simulink model "raspberrypi_multicore_audio_tasks_mapped"  (R2021a)
settings: Solver=FixedStepAuto  StartTime=0.0  StopTime=10.0  RelTol=1e-3  EnableMultiTasking=on
undefined symbols (not defined in the file): plughw
libraries: audiofilters x3, raspberrypiAVlib x2, dspindex x1, audiodynamicrange x1
settings Model: ExplicitPartitioning=on  Creator=The MathWorks, Inc.  LastModifiedBy=The MathWorks, Inc.
settings SolverCC: ConcurrentTasks=on  AlgebraicLoopSolver=TrustRegion  PositivePriorityOrder=on  AutoInsertRateTranBlk=on  InsertRTBMode=Never (minimum delay)
settings OptimizationCC: EnhancedBackFolding=on  PassReuseOutputArgsAs=Individual arguments  ZeroExternalMemoryAtStartup=off  ZeroInternalMemoryAtStartup=off  MaxStackSize=64  OptimizeBlockOrder=speed  DifferentSizesBufferReuse=on  OptimizationCustomize=off  EfficientTunableParamExpr=on
settings DebuggingCC: ParameterTunabilityLossMsg=error  SFMachineParentedDataDiag=warning
settings HardwareCC: ProdBitPerPointer=32  ProdBitPerSizeT=32  ProdBitPerPtrDiffT=32  ProdLargestAtomicInteger=Long  ProdLargestAtomicFloat=Double  ProdWordSize=32  ProdLongLongMode=on  ProdHWDeviceType=ARM Compatible->ARM Cortex
settings RTWCC: SystemTargetFile=ert.tlc  HardwareBoard=Raspberry Pi  TLCOptions="-aInlineSetEventsForThisBaseRateFcn=TLC_FALSE -aSuppressMultiTaskScheduler=TLC_FALSE  -aRateBasedStepFcn=0"  TemplateMakefile=ert_default_tmf  Toolchain=GNU GCC Embedded Linux  BuildConfiguration=Faster Runs
settings CodeAppCC: ForceParamTrailComments=on  IgnoreCustomStorageClasses=off  OperatorAnnotations=on  SimulinkDataObjDesc=on  SFDataObjDesc=on  InsertBlockDesc=on
settings ERTTargetCC: SupportVariableSizeSignals=on

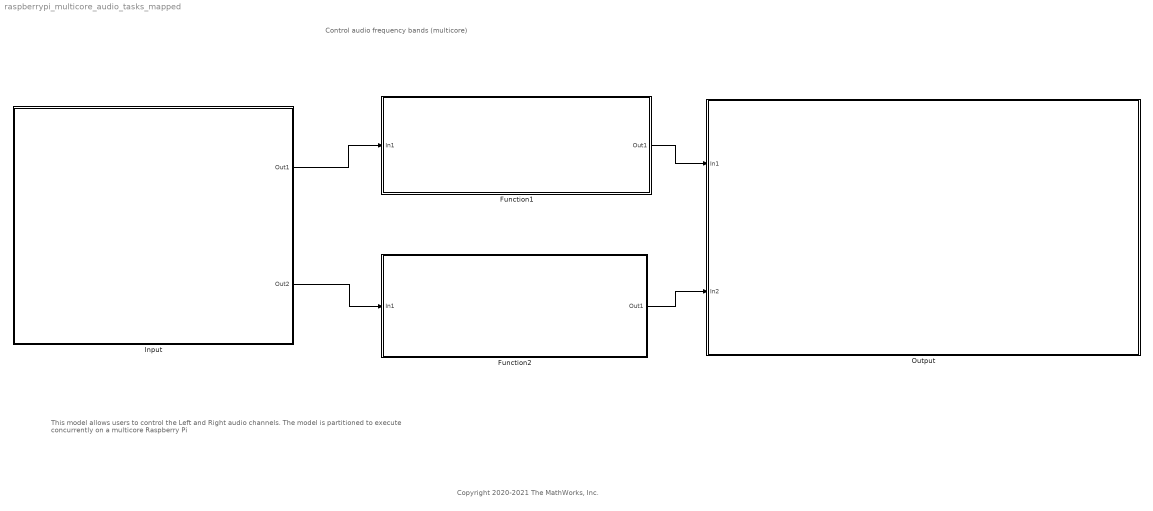
== system raspberrypi_multicore_audio_tasks_mapped ==
  note: This model allows users to control the Left and Right audio channels. The model is partitioned to execute concurrently on a multicore Raspberry Pi
  note: Copyright 2020-2021 The MathWorks, Inc.
  note: Control audio frequency bands (multicore)
  Function1 : Subsystem  TreatAsAtomicUnit=on
  Function2 : Subsystem  TreatAsAtomicUnit=on
  Input : Subsystem  TreatAsAtomicUnit=on
  Output : Subsystem  TreatAsAtomicUnit=on
  wires:
  Input/1(Out1) -> Function1/1(In1)
  Input/2(Out2) -> Function2/1(In1)
  Function1/1(Out1) -> Output/1(In1)
  Function2/1(Out1) -> Output/2(In2)

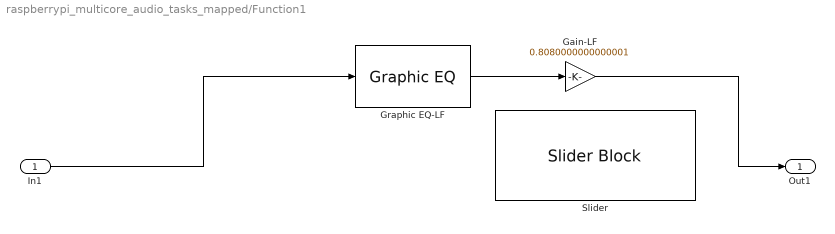
== system raspberrypi_multicore_audio_tasks_mapped/Function1 ==
  In1 : Inport
  Gain-LF : Gain  Gain=0.8080000000000001  OutDataTypeStr=single
  Graphic EQ-LF : audiofilters/Graphic EQ  EQOrder=2  Bandwidth=2/3 octave  Structure=Cascade  Gain_25=12  Gain_31_5=16  Gain_40=16  Gain_50=0  Gain_63=12  Gain_80=0  Gain_100=12  Gain_125=16  Gain_160=12  Gain_200=0  Gain_250=12  Gain_315=-1.200  Gain_400=10.800  Gain_500=6  Gain_630=6  Gain_800=0  Gain_1000=5  Gain_1250=0  Gain_1600=6  Gain_2000=6  Gain_2500=6  Gain_3150=0  Gain_4000=-20  Gain_5000=0  Gain_6300=-20  Gain_8000=-20  Gain_10000=-20  Gain_12500=0  Gain_16000=-20  Gain_20000=0  InheritSampleRate=off  SampleRate=44100  SimulateUsing=Code generation
      settings: SourceProductBaseCode=AU
  Slider : SliderBlock  LabelPosition=Bottom  ScaleMax=1
  Out1 : Outport
  wires:
  Graphic EQ-LF/1 -> Gain-LF/1
  Gain-LF/1 -> Out1/1
  In1/1 -> Graphic EQ-LF/1

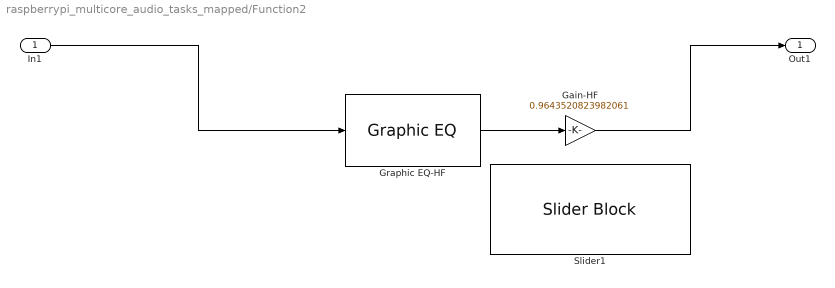
== system raspberrypi_multicore_audio_tasks_mapped/Function2 ==
  In1 : Inport
  Gain-HF : Gain  Gain=0.9643520823982061  OutDataTypeStr=single
  Graphic EQ-HF : audiofilters/Graphic EQ  EQOrder=2  Bandwidth=2/3 octave  Structure=Cascade  Gain_25=-20  Gain_31_5=-20  Gain_40=-20  Gain_50=0  Gain_63=-20  Gain_80=0  Gain_100=-20  Gain_125=-20  Gain_160=-20  Gain_200=0  Gain_250=-20  Gain_315=-1.200  Gain_400=-20  Gain_500=6  Gain_630=-20  Gain_800=0  Gain_1000=0  Gain_1250=0  Gain_1600=3  Gain_2000=6  Gain_2500=3  Gain_3150=0  Gain_4000=0.0  Gain_5000=0  Gain_6300=6  Gain_8000=12  Gain_10000=6  Gain_12500=0  Gain_16000=6  Gain_20000=0  InheritSampleRate=off  SampleRate=44100  SimulateUsing=Code generation
      settings: SourceProductBaseCode=AU
  Slider1 : SliderBlock  LabelPosition=Bottom  ScaleMax=1
  Out1 : Outport
  wires:
  Graphic EQ-HF/1 -> Gain-HF/1
  In1/1 -> Graphic EQ-HF/1
  Gain-HF/1 -> Out1/1

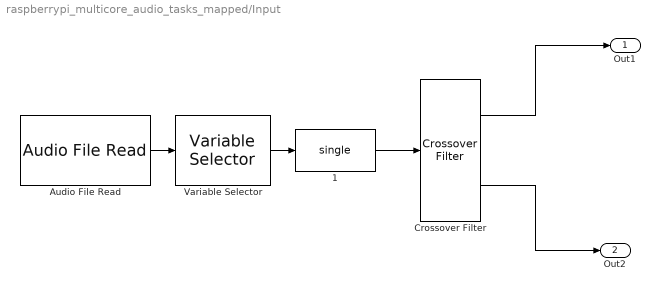
== system raspberrypi_multicore_audio_tasks_mapped/Input ==
  " 1" : DataTypeConversion  OutDataTypeStr=single
  Audio File Read : raspberrypiAVlib/Audio File Read  FileName=guitartune.wav  PlayCount=Inf  OutputEOFIndicator=off  SamplesPerFrame=4410
      settings: SourceProductBaseCode=RASPPI
  Crossover Filter : audiofilters/Crossover Filter  NCrossovers=1  Crossover1Port=off  Crossover1=2.218e+03  Order1Port=off  Order1=8  Crossover2Port=off  Crossover2=800  Order2Port=off  Order2=2  Crossover3Port=off  Crossover3=1500  Order3Port=off  Order3=2  Crossover4Port=off  Crossover4=3000  Order4Port=off  Order4=2  InheritSampleRate=off  SampleRate=44100  SimulateUsing=Code generation
      settings: SourceProductBaseCode=AU
  Variable Selector : dspindex/Variable Selector  NumInputs=1  rowsOrCols=Columns  IdxMode=Fixed  Elements=1  ZerOneIdxMode=One-based  errmode=Clip Index  FillMode=on  FillValues=0
  Out1 : Outport
  Out2 : Outport  Port=2
  wires:
  Audio File Read/1 -> Variable Selector/1
  " 1"/1 -> Crossover Filter/1
  Variable Selector/1 -> " 1"/1
  Crossover Filter/1 -> Out1/1
  Crossover Filter/2 -> Out2/1

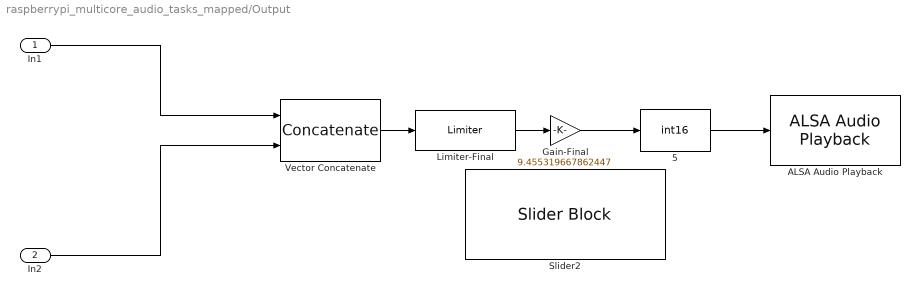
== system raspberrypi_multicore_audio_tasks_mapped/Output ==
  In1 : Inport
  In2 : Inport  Port=2
  " 5" : DataTypeConversion  OutDataTypeStr=int16
  ALSA Audio Playback : raspberrypiAVlib/ALSA Audio Playback  deviceStr=plughw:1,0  sampleRateEnum=44100  queueDuration=0.5  blockPlatform=RASPBERRYPI
      settings: SourceProductBaseCode=RASPPI
  Gain-Final : Gain  Gain=9.455319667862447  OutDataTypeStr=int16
  Limiter-Final : audiodynamicrange/Limiter  ThresholdPort=off  Threshold=-8.0  KneeWidthPort=off  KneeWidth=17.600  AttackTimePort=off  AttackTime=0.9995  ReleaseTimePort=off  ReleaseTime=0.0005  MakeUpGainMode=Property  MakeUpGain=10  InheritSampleRate=off  SampleRate=44100  outputGain=off  SimulateUsing=Code generation
      settings: SourceProductBaseCode=AU
  Slider2 : SliderBlock  LabelPosition=Bottom  ScaleMax=10
  Vector Concatenate : Concatenate  Mode=Multidimensional array  ConcatenateDimension=2
  wires:
  Gain-Final/1 -> " 5"/1
  In2/1 -> Vector Concatenate/2
  In1/1 -> Vector Concatenate/1
  Limiter-Final/1 -> Gain-Final/1
  " 5"/1 -> ALSA Audio Playback/1
  Vector Concatenate/1 -> Limiter-Final/1
